simulink model "exp2M_CSVposRef"  (R2020a)
settings: Solver=FixedStepAuto  StartTime=0.0  StopTime=40  RelTol=1e-3
InitFcn:
  | %Motor1 = Epos4(1,0);
  | %Motor2 = Epos4(2,0);
model workspace (MAT data in the model file):
  NodeID = 1
  OperationMode = 0
  Ts = 0.001
libraries: simulink x2
CloseFcn:
  | %delete(Motor1);
  | %delete(Motor2);
settings Model: DataDictionary=MotorInfo.sldd  Creator=khoi  LastModifiedBy=khoi
settings RTWCC: GenCodeOnly=on

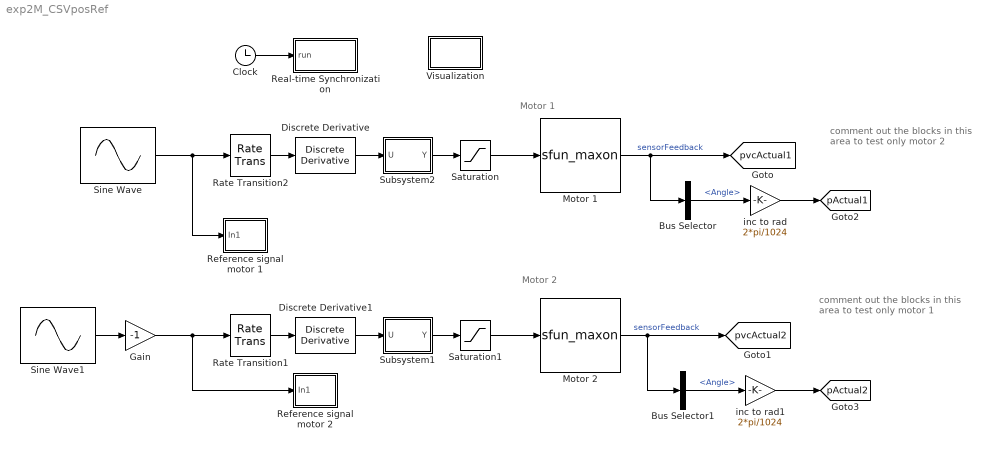
== system exp2M_CSVposRef ==
  note: comment out the blocks in this area to test only motor 1
  note: Motor 2
  note: Motor 1
  note: comment out the blocks in this area to test only motor 2
  Bus Selector : BusSelector  OutputSignals=Angle
  Bus Selector1 : BusSelector  OutputSignals=Angle
  Clock : Clock
  Discrete Derivative : simulink/Discrete/Discrete Derivative  gainval=1.0  ICPrevScaledInput=0.0  OutMin=[]  OutMax=[]  OutDataType=fixdt(1, 16)  OutScaling=2^-10  DoSatur=off
  Discrete Derivative1 : simulink/Discrete/Discrete Derivative  gainval=1.0  ICPrevScaledInput=0.0  OutMin=[]  OutMax=[]  OutDataType=fixdt(1, 16)  OutScaling=2^-10  DoSatur=off
  Gain : Gain  Gain=-1
  Motor 1 : S-Function  FunctionName=sfun_maxon  Parameters=NodeID, DeltaT, OpMode  SFunctionDeploymentMode=off  EnableBusSupport=off  mask{NodeID=1, DeltaT=0.02, OpMode=Cyclic synchronous velocity mode, P_cur=0, I_cur=0, P_pos=0, I_pos=0, D_pos=0, v_posGainFF=0, a_posGainFF=0, P_vel=0, I_vel=0, v_velGainFF=0, a_velGainFF=0, f_velCutoff=0}
      mask prompts: NodeID "Node ID"; DeltaT "Sample time (s)"; OpMode "Operation mode"; P_cur "P gain"; I_cur "I gain"; P_pos "P gain"; I_pos "I gain"; D_pos "D gain"; v_posGainFF "FF velocity gain"; a_posGainFF "FF acceleration gain"; P_vel "P gain"; I_vel "I gain"; v_velGainFF "Feed-forward velocity gain"; a_velGainFF "Feed-forward acceleration gain"; f_velCutoff "Filter cut-off frequency"
      mask TypeOptions OpMode: Cyclic synchronous current (torque) mode | Cyclic synchronous velocity mode | Cyclic synchronous position mode | Profile velocity mode | Profile position mode
      mask DialogControl DescGroupVar Prompt: Motor Parameters
      mask DialogControl DescTextVar Prompt: The block outputs MotorInfo bus signal, which consists of the following variables: angle (increment), speed (rpm), current (mA)
      mask DialogControl Container6 Prompt: Motor
      mask DialogControl Container14 Prompt: Controller Parameters
      mask DialogControl DescTextVar_copy Prompt: This tab is experimental and does not implemented yet. Changing these parameters will not affect the motor performance.
      mask DialogControl Container15 Prompt: Current controller parameter set
      mask DialogControl Container15_copy Prompt: Position controller parameter set
      mask DialogControl Container15_copy_copy Prompt: Velocity controller parameter set
      mask Display:
      | disp('Maxon motor\nHIL');
      | % port_label('input', 1, 'inputSignal');
      | % port_label('output', 1, 'SENSR');
  Motor 2 : S-Function  FunctionName=sfun_maxon  Parameters=NodeID, DeltaT, OpMode  SFunctionDeploymentMode=off  EnableBusSupport=off  mask{NodeID=2, DeltaT=0.02, OpMode=Cyclic synchronous velocity mode, P_cur=0, I_cur=0, P_pos=0, I_pos=0, D_pos=0, v_posGainFF=0, a_posGainFF=0, P_vel=0, I_vel=0, v_velGainFF=0, a_velGainFF=0, f_velCutoff=0}
      mask prompts: NodeID "Node ID"; DeltaT "Sample time (s)"; OpMode "Operation mode"; P_cur "P gain"; I_cur "I gain"; P_pos "P gain"; I_pos "I gain"; D_pos "D gain"; v_posGainFF "FF velocity gain"; a_posGainFF "FF acceleration gain"; P_vel "P gain"; I_vel "I gain"; v_velGainFF "Feed-forward velocity gain"; a_velGainFF "Feed-forward acceleration gain"; f_velCutoff "Filter cut-off frequency"
      mask TypeOptions OpMode: Cyclic synchronous current (torque) mode | Cyclic synchronous velocity mode | Cyclic synchronous position mode | Profile velocity mode | Profile position mode
      mask DialogControl DescGroupVar Prompt: Motor Parameters
      mask DialogControl DescTextVar Prompt: The block outputs MotorInfo bus signal, which consists of the following variables: angle (increment), speed (rpm), current (mA)
      mask DialogControl Container6 Prompt: Motor
      mask DialogControl Container14 Prompt: Controller Parameters
      mask DialogControl DescTextVar_copy Prompt: This tab is experimental and does not implemented yet. Changing these parameters will not affect the motor performance.
      mask DialogControl Container15 Prompt: Current controller parameter set
      mask DialogControl Container15_copy Prompt: Position controller parameter set
      mask DialogControl Container15_copy_copy Prompt: Velocity controller parameter set
      mask Display:
      | disp('Maxon motor\nHIL');
      | % port_label('input', 1, 'inputSignal');
      | % port_label('output', 1, 'SENSR');
  Rate Transition1 : RateTransition  OutPortSampleTime=0.002
  Rate Transition2 : RateTransition  OutPortSampleTime=0.002
  Real-time Synchronization : Subsystem
  Reference signal motor 1 : Subsystem
  Reference signal motor 2 : Subsystem
  Saturation : Saturate  UpperLimit=2000  LowerLimit=-2000
  Saturation1 : Saturate  UpperLimit=2000  LowerLimit=-2000
  Sine Wave : Sin  Amplitude=15  SampleTime=0
  Sine Wave1 : Sin  Amplitude=15  SampleTime=0
  Subsystem1 : Subsystem
      mask Display: disp('To rpm')
  Subsystem2 : Subsystem
      mask Display: disp('To rpm')
  Visualization : Subsystem
  inc to rad : Gain  Gain=2*pi/1024
  inc to rad1 : Gain  Gain=2*pi/1024
  tag scope: pActual1=global, pActual2=global, pvcActual1=global, pvcActual2=global
  wires:
  Clock/1 -> Real-time Synchronization/1(run)
  Motor 2/1 -> [pvcActual2], Bus Selector1/1  "sensorFeedback"
  Saturation1/1 -> Motor 2/1
  Motor 1/1 -> [pvcActual1], Bus Selector/1  "sensorFeedback"
  Bus Selector/1 -> inc to rad/1  "<Angle>"
  Bus Selector1/1 -> inc to rad1/1  "<Angle>"
  inc to rad/1 -> [pActual1]
  inc to rad1/1 -> [pActual2]
  Sine Wave/1 -> Reference signal motor 1/1(In1), Rate Transition2/1
  Rate Transition2/1 -> Discrete Derivative/1
  Saturation/1 -> Motor 1/1
  Discrete Derivative/1 -> Subsystem2/1(U)
  Subsystem2/1(Y) -> Saturation/1
  Subsystem1/1(Y) -> Saturation1/1
  Discrete Derivative1/1 -> Subsystem1/1(U)
  Rate Transition1/1 -> Discrete Derivative1/1
  Sine Wave1/1 -> Gain/1
  Gain/1 -> Reference signal motor 2/1(In1), Rate Transition1/1

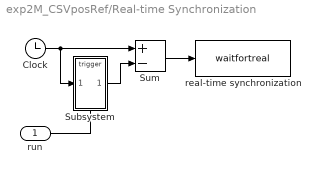
== system exp2M_CSVposRef/Real-time Synchronization ==
  run : Inport
  Clock : Clock
  Subsystem : Subsystem  TreatAsAtomicUnit=on
  Sum : Sum  Inputs=+-  InputSameDT=on  SaturateOnIntegerOverflow=on  OutDataTypeStr=Inherit: Same as first input
  real-time synchronization : MATLABFcn  MATLABFcn=waitfortreal  OutputDimensions=0
  wires:
  Clock/1 -> Subsystem/1(In), Sum/1
  Subsystem/1(Out) -> Sum/2
  Sum/1 -> real-time synchronization/1
  run/1 -> Subsystem/Trigger

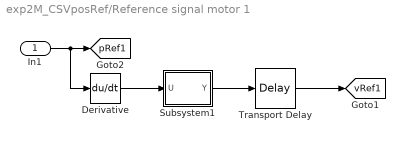
== system exp2M_CSVposRef/Reference signal motor 1 ==
  In1 : Inport
  Derivative : Derivative
  Subsystem1 : Subsystem
      mask Display: disp('To rpm')
  Transport Delay : TransportDelay  DelayTime=0.1
  tag scope: pRef1=global, vRef1=global
  wires:
  Subsystem1/1(Y) -> Transport Delay/1
  Derivative/1 -> Subsystem1/1(U)
  In1/1 -> Derivative/1, [pRef1]
  Transport Delay/1 -> [vRef1]

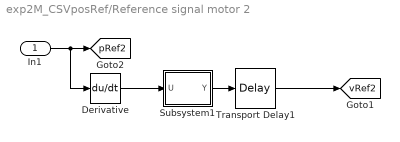
== system exp2M_CSVposRef/Reference signal motor 2 ==
  In1 : Inport
  Derivative : Derivative
  Subsystem1 : Subsystem
      mask Display: disp('To rpm')
  Transport Delay1 : TransportDelay  DelayTime=0.1
  tag scope: pRef2=global, vRef2=global
  wires:
  Subsystem1/1(Y) -> Transport Delay1/1
  In1/1 -> [pRef2], Derivative/1
  Derivative/1 -> Subsystem1/1(U)
  Transport Delay1/1 -> [vRef2]

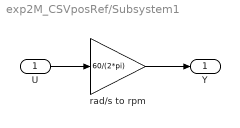
== system exp2M_CSVposRef/Subsystem1 ==
  U : Inport
  rad/s to rpm : Gain  Gain=60/(2*pi)
  Y : Outport
  wires:
  rad/s to rpm/1 -> Y/1
  U/1 -> rad/s to rpm/1

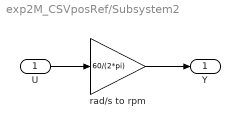
== system exp2M_CSVposRef/Subsystem2 ==
  U : Inport
  rad/s to rpm : Gain  Gain=60/(2*pi)
  Y : Outport
  wires:
  U/1 -> rad/s to rpm/1
  rad/s to rpm/1 -> Y/1

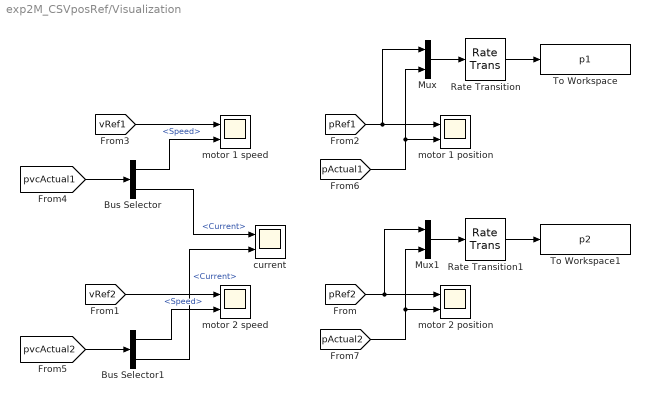
== system exp2M_CSVposRef/Visualization ==
  Bus Selector : BusSelector  OutputSignals=Speed,Current
  Bus Selector1 : BusSelector  OutputSignals=Speed,Current
  Mux : Mux  Inputs=2
  Mux1 : Mux  Inputs=2
  Rate Transition : RateTransition  OutPortSampleTime=0.02
  Rate Transition1 : RateTransition  OutPortSampleTime=0.02
  To Workspace : ToWorkspace  VariableName=p1  SaveFormat=Timeseries  SampleTime=-1
  To Workspace1 : ToWorkspace  VariableName=p2  SaveFormat=Timeseries  SampleTime=-1
  current : Scope  NumInputPorts=2
  motor 1 position : Scope  NumInputPorts=2
  motor 1 speed : Scope  NumInputPorts=2
  motor 2 position : Scope  NumInputPorts=2
  motor 2 speed : Scope  NumInputPorts=2
  wires:
  [pActual1] -> Mux/2, motor 1 position/2
  [vRef2] -> motor 2 speed/1
  [pvcActual2] -> Bus Selector1/1
  [pvcActual1] -> Bus Selector/1
  [pRef1] -> Mux/1, motor 1 position/1
  [vRef1] -> motor 1 speed/1
  [pActual2] -> Mux1/2, motor 2 position/2
  Bus Selector1/1 -> motor 2 speed/2  "<Speed>"
  Bus Selector/1 -> motor 1 speed/2  "<Speed>"
  Bus Selector/2 -> current/1  "<Current>"
  Bus Selector1/2 -> current/2  "<Current>"
  Rate Transition/1 -> To Workspace/1
  Mux/1 -> Rate Transition/1
  Mux1/1 -> Rate Transition1/1
  Rate Transition1/1 -> To Workspace1/1
  [pRef2] -> Mux1/1, motor 2 position/1

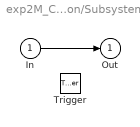
== system exp2M_CSVposRef/Real-time Synchronization/Subsystem ==
  In : Inport
  Trigger : TriggerPort  VariantControl=(inherit)
  Out : Outport  InitialOutput=0
  wires:
  In/1 -> Out/1

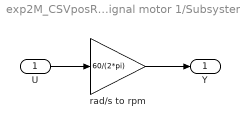
== system exp2M_CSVposRef/Reference signal motor 1/Subsystem1 ==
  U : Inport
  rad/s to rpm : Gain  Gain=60/(2*pi)
  Y : Outport
  wires:
  rad/s to rpm/1 -> Y/1
  U/1 -> rad/s to rpm/1

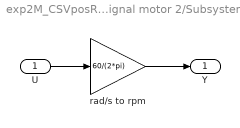
== system exp2M_CSVposRef/Reference signal motor 2/Subsystem1 ==
  U : Inport
  rad/s to rpm : Gain  Gain=60/(2*pi)
  Y : Outport
  wires:
  rad/s to rpm/1 -> Y/1
  U/1 -> rad/s to rpm/1
